simulink model "Three_phase_120_degree_inverter"  (R2024b)
settings: Solver=VariableStepAuto  StartTime=0.0  StopTime=10.0  RelTol=1e-3
libraries: spsIGBTDiodeLib x6, spsVoltageMeasurementLib x6, spsSeriesRLCBranchLib x3, spsDCVoltageSourceLib x1, spsGroundLib x1, sps_lib x1
settings Model: Creator=HARSH  LastModifiedBy=HARSH

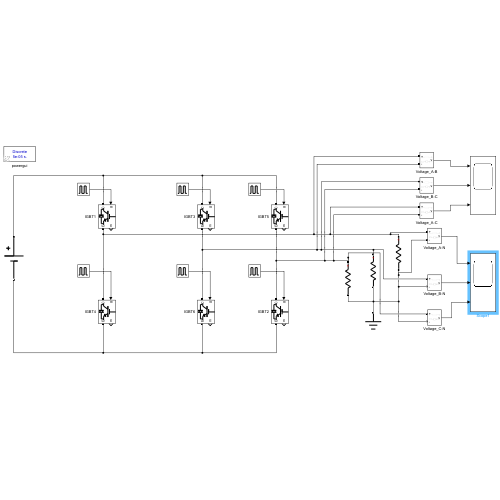
[thumbnail: Simulink's stored preview of the top-level diagram]
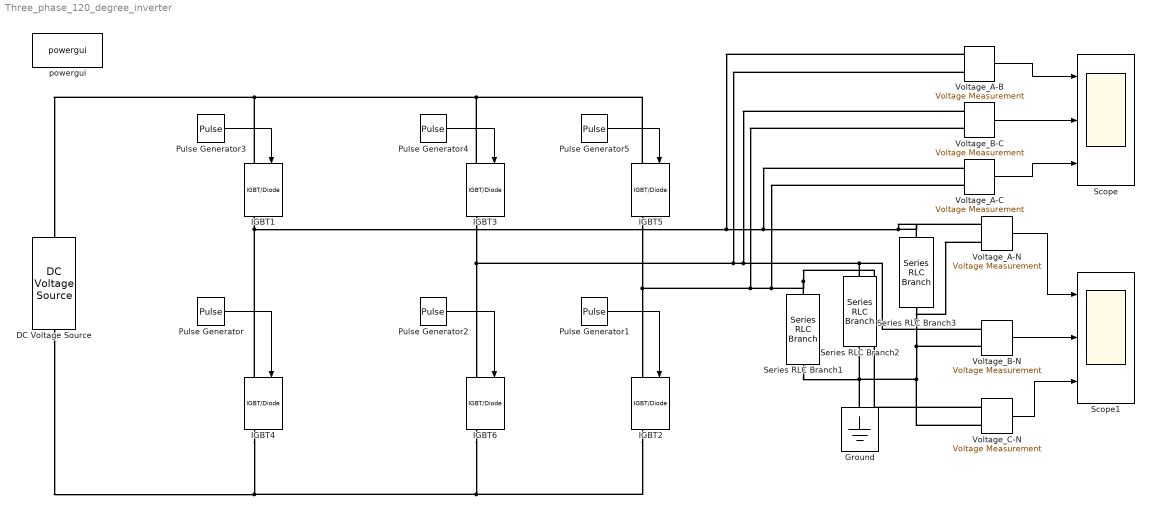
== system Three_phase_120_degree_inverter ==
  DC Voltage Source : spsDCVoltageSourceLib/DC Voltage Source  Amplitude=100  Measurements=None
  Ground : spsGroundLib/Ground  LConnTagsString=a
  IGBT{1..6} (6 alike) : spsIGBTDiodeLib/IGBT//Diode  Ron=1e-3  Rs=1e5  Cs=inf  Measurements=on
  Pulse Generator : DiscretePulseGenerator  PulseType=Time based  Period=0.02  PulseWidth=100/3  PhaseDelay=0.02*180/360
  Pulse Generator1 : DiscretePulseGenerator  PulseType=Time based  Period=0.02  PulseWidth=100/3  PhaseDelay=0.02*60/360
  Pulse Generator2 : DiscretePulseGenerator  PulseType=Time based  Period=0.02  PulseWidth=100/3  PhaseDelay=0.02*300/360
  Pulse Generator3 : DiscretePulseGenerator  PulseType=Time based  Period=0.02  PulseWidth=100/3
  Pulse Generator4 : DiscretePulseGenerator  PulseType=Time based  Period=0.02  PulseWidth=100/3  PhaseDelay=0.02*120/360
  Pulse Generator5 : DiscretePulseGenerator  PulseType=Time based  Period=0.02  PulseWidth=100/3  PhaseDelay=0.02*240/360
  Scope : Scope  NumInputPorts=3
  Scope1 : Scope  NumInputPorts=3
  Series RLC Branch1 : spsSeriesRLCBranchLib/Series RLC Branch  LConnTagsString=__new0  RConnTagsString=__new0  BranchType=R  Resistance=10  Inductance=50e-3  SetiL0=off  InitialCurrent=0  Capacitance=1e-6  Setx0=off  InitialVoltage=0  Measurements=None
  Series RLC Branch2 : spsSeriesRLCBranchLib/Series RLC Branch  LConnTagsString=__new0  RConnTagsString=__new0  BranchType=R  Resistance=10  Inductance=50e-3  SetiL0=off  InitialCurrent=0  Capacitance=1e-6  Setx0=off  InitialVoltage=0  Measurements=None
  Series RLC Branch3 : spsSeriesRLCBranchLib/Series RLC Branch  LConnTagsString=__new0  RConnTagsString=__new0  BranchType=R  Resistance=10  Inductance=50e-3  SetiL0=off  InitialCurrent=0  Capacitance=1e-6  Setx0=off  InitialVoltage=0  Measurements=None
  Voltage_A-B : spsVoltageMeasurementLib/Voltage Measurement  PhasorSimulation=off  OutputType=Complex  PSBequivalent=0
  Voltage_A-C : spsVoltageMeasurementLib/Voltage Measurement  PhasorSimulation=off  OutputType=Complex  PSBequivalent=0
  Voltage_A-N : spsVoltageMeasurementLib/Voltage Measurement  PhasorSimulation=off  OutputType=Complex  PSBequivalent=0
  Voltage_B-C : spsVoltageMeasurementLib/Voltage Measurement  PhasorSimulation=off  OutputType=Complex  PSBequivalent=0
  Voltage_B-N : spsVoltageMeasurementLib/Voltage Measurement  PhasorSimulation=off  OutputType=Complex  PSBequivalent=0
  Voltage_C-N : spsVoltageMeasurementLib/Voltage Measurement  PhasorSimulation=off  OutputType=Complex  PSBequivalent=0
  powergui : sps_lib/powergui  Priority=1  SimulationMode=Discrete  SampleTime=50e-6  frequency=60  Iterations=50  frequencyindice=0  Pbase=100e6  ErrMax=1e-4  UnitsV=kV  UnitsW=MW  buscounter=0  FunctionMessages=off  echomessages=off  EnableUseOfTLC=off  CurrentSourceSwitches=off  DisableSnubberDevices=off  DisableRonSwitches=off  DisableVfSwitches=off  DisplayEquations=off  AutomaticDiscreteSolvers=off  SolverType=Tustin/Backward Euler (TBE)  Interpol=off  ExternalGateDelay=off  methode=off  Ts=100  x0status=blocks  SPID=on  SwTol=0  HookPort=off  NonlinearTolerance=1e-4  nMaxIteration=100  ContinueOnMaxIteration=off  RestoreLinks=warning  ResistiveCurrentMeasurement=off  Frange=[0:2:500]  Ylog=off  Xlog=on  ShowGrid=off  save=off  variable=ZData  structure=0  ZoomFFT=off  StartTime=0.0  cycles=1  DisplayStyle=1  fundamental=60  FreqAxis=off  MaxFrequency=1000  frequencyindicesteady=1  RmsSteady=1  display=off
  wires:
  Pulse Generator4/1 -> IGBT3/1
  Pulse Generator/1 -> IGBT4/1
  Pulse Generator5/1 -> IGBT5/1
  Pulse Generator3/1 -> IGBT1/1
  Pulse Generator2/1 -> IGBT6/1
  Voltage_B-C/1 -> Scope/2
  Voltage_B-N/1 -> Scope1/2
  Voltage_A-N/1 -> Scope1/1
  Voltage_C-N/1 -> Scope1/3
  Voltage_A-C/1 -> Scope/3
  Voltage_A-B/1 -> Scope/1
  Pulse Generator1/1 -> IGBT2/1
  connections:
  IGBT3/LConn1 -- DC Voltage Source/RConn1 -- IGBT1/LConn1 -- IGBT5/LConn1
  IGBT3/RConn1 -- Voltage_B-C/LConn1 -- Voltage_B-N/LConn1 -- Series RLC Branch2/LConn1 -- Voltage_A-B/LConn2 -- IGBT6/LConn1
  IGBT1/RConn1 -- IGBT4/LConn1 -- Voltage_A-C/LConn1 -- Series RLC Branch3/LConn1 -- Voltage_A-N/LConn1 -- Voltage_A-B/LConn1
  IGBT4/RConn1 -- IGBT2/RConn1 -- IGBT6/RConn1 -- DC Voltage Source/LConn1
  IGBT5/RConn1 -- Voltage_A-C/LConn2 -- Voltage_C-N/LConn1 -- Series RLC Branch1/LConn1 -- Voltage_B-C/LConn2 -- IGBT2/LConn1
  Ground/LConn1 -- Series RLC Branch3/RConn1 -- Voltage_A-N/LConn2 -- Voltage_B-N/LConn2 -- Voltage_C-N/LConn2 -- Series RLC Branch1/RConn1 -- Series RLC Branch2/RConn1
